simulink library "thermochemical"  (R2017b)
settings: Solver=VariableStepAuto  StartTime=0.0  StopTime=10.0  RelTol=1e-3
values from neighbouring files (symbols this model uses):
  c = conversion_factors()    [blk_clausius_clapeyron.m]    (also in blk_clausius_clapeyron_no_popup.m; blk_cold_room_closed_dry_air.m; blk_reactor_BaCl2_NH3_no_walls.m; blk_reactor_BaCl2_NH3_no_walls_state_space.m)
  cp = metal.cp    [blk_wall_simple.m]    (also in get_metal_properties.m = 390)
  fluid = get_param(blk,'fluid')    [blk_thermodynamic_properties_nonsaturated.m]    (also in blk_thermodynamic_properties_nonsaturated_interpreted.m; blk_thermodynamic_properties_saturated.m; blk_thermodynamic_properties_saturated_interpreted.m; blk_thermodynamic_properties_saturated_mix.m)
  gas = get_material_properties(x.gasName)    [blk_reactor_BaCl2_NH3_cylindrical_no_walls_fun1.m]
  h = get_param(gcb,'ObjectParameters')    [get_param_eval.m]
  rho = metal.rho    [blk_wall_simple.m]    (also in get_metal_properties.m = 8940)
  s = solve(eq,dx,'ReturnConditions',true)    [LMTD_inv.m]    (also in blk_wall_simple.m = get_param_eval(blk,'s'))
  u_gas_at_T_ref = -R * T_ref    [blk_reactor_BaCl2_NH3_no_walls.m]    (also in blk_reactor_BaCl2_NH3_no_walls_state_space.m)
undefined symbols (not defined in the file or in its folder): b_motor, BaCl2, beta, CoolProp, cP_binder, cP_gas, cP_s0, cv, dh_r_0, ENG, heat_exchanger_epsilonNTU_inv_simulink, heat_exchanger_epsilonNTU_simulink, J_motor, K_cin, kappa, Km_motor, La_motor, lookup2D_BreakPoint2, M_binder, N_binder, N_gas_free_volume_init, N_salt, NH3, nh3_v3, nu, P, phase, PID_D_motor, PID_I_motor, PID_P_motor, Ra_motor, Reactor_phase, T, T1, T2, T_init, Tr_init, Tr_ref, U_binder_at_Tr_ref, U_salt_at_X0_Tr_ref, Ur_init, V_void, Valve_regime, Vmax_motor, w_init_motor, X_init
libraries: thermochemical x247, simulink x54, dspsigops x3
(part 12 of 12)

== system thermochemical/Reactors/Reactor, BaCl2//NH3, state-space form, [Tr, Ng, X] as state variables, no algebraic loops, real gas in void volume, ideal gas in salt/Reactor, BaCl2//NH3, no walls, state-space form, [Tr, Ng, X] as state variables, no algebraic loops, real gas in void volume, ideal gas in salt/Reactor, no walls, state space form/Reactor state-space functions/f1/f3/Reaction kinetic, differential equation ==
  note: Desorption
  note: Synthesis
  In1 : Inport
  In2 : Inport  Port=2
  In3 : Inport  Port=3
  3 : Constant
  Clausius-Clapeyron : thermochemical/Thermodynamic fluid properties/Clausius-Clapeyron  sel_1=P(T)  sel_2=BaCl2/NH3
      settings: SourceProductName=@ Thermochemical
  Divide1 : Product  Inputs=/*
  Gain15 : Gain  Gain=K_cin
  Product6 : Product
  Relay : Relay  OnSwitchValue=P_dead_zone  OffSwitchValue=-P_dead_zone  OffOutputValue=-1
  Sum16 : Sum  Inputs=+-
  Sum17 : Sum  Inputs=+-|
  Switch : Switch  Criteria=u2 > Threshold
  Out2 : Outport
  wires:
  Sum17/1 -> Switch/1  "1 - X"
  Divide1/1 -> Gain15/1
  Switch/1 -> Product6/2
  In2/1 -> Sum16/1, Divide1/1  "P (bar)"
  Product6/1 -> Out2/1  "dX/dt"
  3/1 -> Sum17/1
  Gain15/1 -> Product6/1
  Clausius-Clapeyron/1 -> Sum16/2  "P_equilb (bar)"
  Sum16/1 -> Relay/1, Divide1/2  "dP"
  In1/1 -> Clausius-Clapeyron/1  "T(K)"
  Relay/1 -> Switch/2
  In3/1 -> Sum17/2, Switch/3  "X (0..1)"

== system thermochemical/Reactors/Reactor, BaCl2//NH3, state-space form, [Tr, Ng, X] as state variables, no algebraic loops, real gas in void volume, real gas in salt/Reactor, BaCl2//NH3, no walls, state-space form, [Tr, Ng, X] as state variables, no algebraic loops, real gas in void volume, real gas in salt/Reactor, no walls, state space form/Reactor state-space functions/f1/f3/Reaction kinetic, differential equation ==
  note: Synthesis
  note: Desorption
  In1 : Inport
  In2 : Inport  Port=2
  In3 : Inport  Port=3
  3 : Constant
  Clausius-Clapeyron : thermochemical/Thermodynamic fluid properties/Clausius-Clapeyron  sel_1=P(T)  sel_2=BaCl2/NH3
      settings: SourceProductName=@ Thermochemical
  Divide1 : Product  Inputs=/*
  Gain15 : Gain  Gain=K_cin
  Product6 : Product
  Relay : Relay  OnSwitchValue=P_dead_zone  OffSwitchValue=-P_dead_zone  OffOutputValue=-1
  Sum16 : Sum  Inputs=+-
  Sum17 : Sum  Inputs=+-|
  Switch : Switch  Criteria=u2 > Threshold
  Out2 : Outport
  wires:
  In3/1 -> Switch/3, Sum17/2  "X (0..1)"
  Relay/1 -> Switch/2
  In1/1 -> Clausius-Clapeyron/1  "T(K)"
  Sum16/1 -> Divide1/2, Relay/1  "dP"
  Clausius-Clapeyron/1 -> Sum16/2  "P_equilb (bar)"
  Gain15/1 -> Product6/1
  3/1 -> Sum17/1
  Product6/1 -> Out2/1  "dX/dt"
  In2/1 -> Divide1/1, Sum16/1  "P (bar)"
  Switch/1 -> Product6/2
  Divide1/1 -> Gain15/1
  Sum17/1 -> Switch/1  "1 - X"

== system thermochemical/Reactors/Reactor, BaCl2//NH3, state-space form, [Ur, Ng, X] as state variables, no algebraic loops, ideal gas in void volume, ideal gas in salt/Reactor, BaCl2//NH3, no walls, state-space form, [Ur, Ng, X] as state variables, no algebraic loops, ideal gas in void volume, ideal gas in salt/Reactor, no walls, state space form/Reactor state-space functions/f3/f3/Reaction kinetic, differential equation ==
  note: Desorption
  note: Synthesis
  In1 : Inport
  In2 : Inport  Port=2
  In3 : Inport  Port=3
  3 : Constant
  Clausius-Clapeyron : thermochemical/Thermodynamic fluid properties/Clausius-Clapeyron  sel_1=P(T)  sel_2=BaCl2/NH3
      settings: SourceProductName=@ Thermochemical
  Divide1 : Product  Inputs=/*
  Gain15 : Gain  Gain=K_cin
  Product6 : Product
  Relay : Relay  OnSwitchValue=P_dead_zone  OffSwitchValue=-P_dead_zone  OffOutputValue=-1
  Sum16 : Sum  Inputs=+-
  Sum17 : Sum  Inputs=+-|
  Switch : Switch  Criteria=u2 > Threshold
  Out2 : Outport
  wires:
  Sum17/1 -> Switch/1  "1 - X"
  Divide1/1 -> Gain15/1
  Switch/1 -> Product6/2
  In2/1 -> Sum16/1, Divide1/1  "P (bar)"
  Product6/1 -> Out2/1  "dX/dt"
  3/1 -> Sum17/1
  Gain15/1 -> Product6/1
  Clausius-Clapeyron/1 -> Sum16/2  "P_equilb (bar)"
  Sum16/1 -> Relay/1, Divide1/2  "dP"
  In1/1 -> Clausius-Clapeyron/1  "T(K)"
  Relay/1 -> Switch/2
  In3/1 -> Sum17/2, Switch/3  "X (0..1)"

== matlab function thermochemical/Heat exchangers/Heat Exchanger, e-NTU method (epsilon input) Loop 2: water/Subsystem/NTU as a function of flow configuration/MATLAB Function ==
  data: epsilon input double; NTU output double; Cr input double; flowType_numeric input double
function NTU = fcn(epsilon, Cr, flowType_numeric)

switch(flowType_numeric)
    case 0
        flowType = 'Counter-flow';
    case 1
        flowType = 'Parallel-flow';
    case 2
        flowType = 'Cross-flow, both unmixed';
    case 3
        flowType = 'Cross-flow, both mixed';
    case 4
        flowType = 'Cross-flow, Cmax mixed, Cmin unmixed';
    case 5
        flowType = 'Cross-flow, Cmin mixed, Cmax unmixed';
    case 6
        flowType = 'Condensation/evaporation';
    otherwise
        error('Wrong flow type or flow type not implemented.')
end

NTU = double(heat_exchanger_NTU_function(epsilon, Cr, flowType));

== matlab function thermochemical/Heat exchangers/Heat Exchanger, e-NTU method (UA input) Loop 2: water/Subsystem/NTU as a function of flow configuration/MATLAB Function ==
  data: NTU input double; epsilon output double; Cr input double; flowType_numeric input double
function epsilon = fcn(NTU, Cr, flowType_numeric)

switch(flowType_numeric)
    case 0
        flowType = 'Counter-flow';
    case 1
        flowType = 'Parallel-flow';
    case 2
        flowType = 'Cross-flow, both unmixed';
    case 3
        flowType = 'Cross-flow, both mixed';
    case 4
        flowType = 'Cross-flow, Cmax mixed, Cmin unmixed';
    case 5
        flowType = 'Cross-flow, Cmin mixed, Cmax unmixed';
    case 6
        flowType = 'Condensation/evaporation';
    otherwise
        error('Wrong flow type or flow type not implemented.')
end

epsilon = double(heat_exchanger_epsilon_function(NTU, Cr, flowType));
